simulink model "gm_uz_pmsm_model_9ph_21b_all_double"  (R2021b)
settings: Solver=FixedStepAuto  StartTime=0.0  StopTime=0.8  RelTol=1e-3
PreLoadFcn:
  | uz_pmsm_model_9ph_init_parameter
undefined symbols (not defined in the file or in its folder): a, b, c, friction_coefficient, inertia, k_i_d, k_i_q, k_p_d, k_p_q, Kpd, L_d, L_o1, L_o2, L_q, L_x1, L_x2, L_y1, L_y2, L_zero, polepair, psi_pm, R_1, static_friction_torque, Tnd, ts
libraries: hdlsllib x90, simulink x32, hdlmdlgenlib x17, dspsigops x7, slpidlib x2, spsAlphaBetaZerotodq0Lib x1, pid_lib x1, spsdq0toAlphaBetaZeroLib x1
(part 3 of 6)

== system gm_uz_pmsm_model_9ph_21b_all_double/uz_pmsm_model_9ph/dq_model_9ph/Wrapped State DTI ==
  note: https://de.mathworks.com/help/releases/R2021a/hdlcoder/ug/troubleshoot-generate-implementation-model-from-simscape-pmsm.html?searchHighlight=troubleshoot-generate-implementation-model-from-simscape-pmsm&s_tid=doc_srchtitle
  Angular Speed : Inport
  polepair : Inport  Port=2
  reset : Inport  Port=3
  Compare To Constant : simulink/Logic and Bit Operations/Compare To Constant  relop=>=  const=single(pi)  OutDataTypeStr=boolean
  Compare To Constant1 : simulink/Logic and Bit Operations/Compare To Constant  relop=<  const=single(-pi)  OutDataTypeStr=boolean
  Constant : Constant  Value=double(2*pi)  SampleTime=-1
  Delay1 : Delay  DelayLength=1  ExternalReset=Level
      settings: InputPortMap=u0,r5
  Gain : Gain  Gain=ts
  Product : Product
  Sum : Sum  Inputs=|++
  Sum1 : Sum  Inputs=|-+
  Sum2 : Sum  Inputs=|++
  Switch : Switch  Criteria=u2 > Threshold
  Switch1 : Switch  Criteria=u2 > Threshold
  Angular Position : Outport
  wires:
  Compare To Constant1/1 -> Switch1/2
  Delay1/1 -> Sum/1, Angular Position/1
  Constant/1 -> Sum2/1, Sum1/1
  Sum2/1 -> Switch1/1
  Switch1/1 -> Delay1/1  "Angular Position"
  Switch/1 -> Sum2/2, Compare To Constant1/1, Switch1/3
  Compare To Constant/1 -> Switch/2
  Sum/1 -> Compare To Constant/1, Sum1/2, Switch/3
  Sum1/1 -> Switch/1
  Gain/1 -> Sum/2
  reset/1 -> Delay1/2
  Product/1 -> Gain/1
  Angular Speed/1 -> Product/1
  polepair/1 -> Product/2

== system gm_uz_pmsm_model_9ph_21b_all_double/uz_pmsm_model_9ph/dq_model_9ph/mechanical_system ==
  note: load torque negative!!!
  note: This delay breaks the algebraic loop between mechanical and electrical system.
      | Introduces a delay of 500ns.
  reset : Inport
  M_Mi : Inport  Port=2
  reciprocal_J : Inport  Port=3
  load_torque : Inport  Port=4
  Delay : Delay  DelayLength=1
  Product11 : Product
  Sum1 : Sum  Inputs=|++
  integrator : Subsystem
  omega_mech : Outport
  wires:
  reciprocal_J/1 -> Product11/1
  Sum1/1 -> Product11/2
  load_torque/1 -> Sum1/2
  M_Mi/1 -> Delay/1
  Delay/1 -> Sum1/1
  integrator/1(outt) -> omega_mech/1
  Product11/1 -> integrator/1(in)
  reset/1 -> integrator/2(reset)

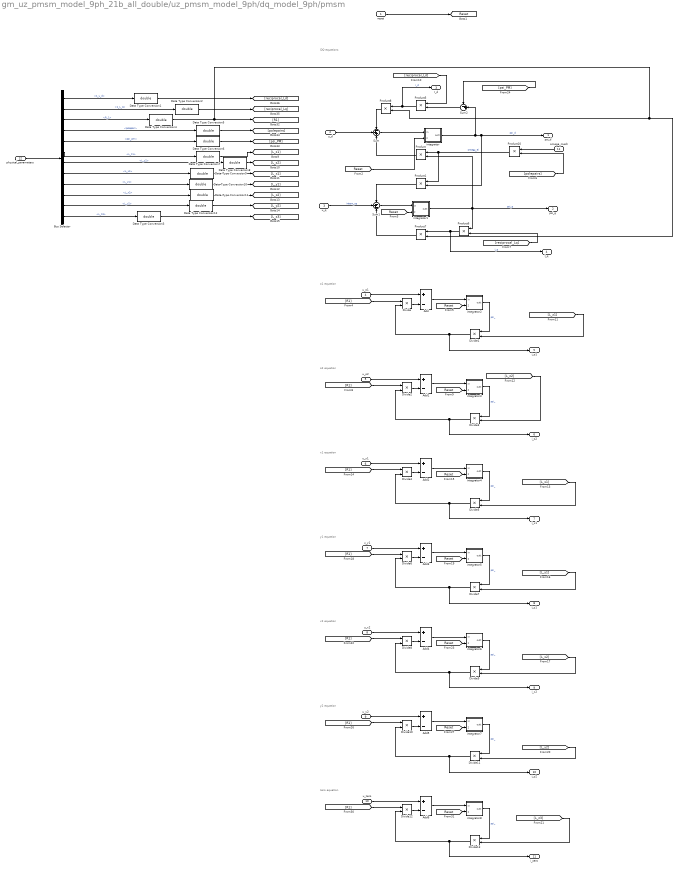
== system gm_uz_pmsm_model_9ph_21b_all_double/uz_pmsm_model_9ph/dq_model_9ph/pmsm ==
  note: o1 equation
  note: DQ equations
  note: o2 equation
  note: x1 equation
  note: y1 equation
  note: x2 equation
  note: y2 equation
  note: zero equation
  reset : Inport
  u_d : Inport  Port=2
  u_q : Inport  Port=3
  u_o1 : Inport  Port=4
  u_o2 : Inport  Port=5
  u_x1 : Inport  Port=6
  u_y1 : Inport  Port=7
  u_x2 : Inport  Port=8
  u_y2 : Inport  Port=9
  u_zero : Inport  Port=10
  omega_mech : Inport  Port=11
  physical_parameters : Inport  Port=12
  Add{,1..6} (7 alike) : Sum  Inputs=+-
  Bus Selector : BusSelector  OutputSignals=1_L_d,1_L_q,R_1,polepair,psi_pm,L_z1,L_z2,L_x1,L_y1,L_x2,L_y2,L_z3
  Data Type Conversion{1..12} (12 alike) : DataTypeConversion  OutDataTypeStr=double  RndMeth=Nearest
  Divide{,1..13} (14 alike) : Product  Inputs=**
  Product{,1,5..8,10} (7 alike) : Product
  Sum : Sum  Inputs=-++
  Sum1 : Sum  Inputs=-+-
  Sum2 : Sum  Inputs=-+|
  integrator : Subsystem
  integrator1 : Subsystem
  integrator2 : Subsystem
  integrator3 : Subsystem
  integrator4 : Subsystem
  integrator5 : Subsystem
  integrator6 : Subsystem
  integrator7 : Subsystem
  integrator8 : Subsystem
  psi_d : Outport
  psi_q : Outport  Port=2
  I_d : Outport  Port=3
  I_q : Outport  Port=4
  i_o1 : Outport  Port=5
  i_o2 : Outport  Port=6
  i_x1 : Outport  Port=7
  i_y1 : Outport  Port=8
  i_x2 : Outport  Port=9
  i_y2 : Outport  Port=10
  i_zero : Outport  Port=11
  tag scope: Reset=global
  wires:
  omega_mech/1 -> Product10/1
  u_q/1 -> Sum1/2  "intern_uq"
  Product/1 -> Sum/3
  Product5/1 -> I_d/1, Product8/1  "I_d"
  [reciprocal_Ld] -> Product5/1
  integrator1/1(outt) -> psi_q/1, Product/2, Product6/1  "psi_q"
  Product1/1 -> Sum1/1
  [psi_PM] -> Sum2/1
  Product6/1 -> I_q/1, Product7/1  "I_q"
  Product10/1 -> Product1/1, Product/1  "omega_el"
  integrator/1(outt) -> Sum2/2, psi_d/1, Product1/2  "psi_d"
  Sum2/1 -> Product5/2
  Product8/1 -> Sum/1
  [reciprocal_Lq] -> Product6/2
  Product7/1 -> Sum1/3
  reset/1 -> [Reset]
  [Reset] -> integrator/2(reset)
  [Reset] -> integrator1/2(reset)
  [Reset] -> integrator2/2(reset)
  [L_z1] -> Divide1/2
  u_o1/1 -> Add/1
  Divide1/1 -> i_o1/1, Divide/2
  Divide/1 -> Add/2
  [R1] -> Divide/1
  integrator2/1(outt) -> Divide1/1  "psi_"
  integrator3/1(outt) -> Divide3/1  "psi_"
  [R1] -> Divide2/1
  Divide2/1 -> Add1/2
  Divide3/1 -> i_o2/1, Divide2/2
  u_o2/1 -> Add1/1
  [L_z2] -> Divide3/2
  [Reset] -> integrator3/2(reset)
  [Reset] -> integrator4/2(reset)
  u_x1/1 -> Add2/1
  Divide5/1 -> i_x1/1, Divide4/2
  Divide4/1 -> Add2/2
  [R1] -> Divide4/1
  integrator4/1(outt) -> Divide5/1  "psi_"
  integrator5/1(outt) -> Divide7/1  "psi_"
  [R1] -> Divide6/1
  Divide6/1 -> Add3/2
  Divide7/1 -> i_y1/1, Divide6/2
  u_y1/1 -> Add3/1
  [Reset] -> integrator5/2(reset)
  [Reset] -> integrator6/2(reset)
  u_x2/1 -> Add4/1
  Divide9/1 -> i_x2/1, Divide8/2
  Divide8/1 -> Add4/2
  [R1] -> Divide8/1
  integrator6/1(outt) -> Divide9/1  "psi_"
  integrator7/1(outt) -> Divide11/1  "psi_"
  [R1] -> Divide10/1
  Divide10/1 -> Add5/2
  Divide11/1 -> i_y2/1, Divide10/2
  u_y2/1 -> Add5/1
  [Reset] -> integrator7/2(reset)
  [Reset] -> integrator8/2(reset)
  u_zero/1 -> Add6/1
  Divide13/1 -> i_zero/1, Divide12/2
  Divide12/1 -> Add6/2
  [R1] -> Divide12/1
  integrator8/1(outt) -> Divide13/1  "psi_"
  Bus Selector/1 -> Data Type Conversion1/1  "<1_L_d>"
  Bus Selector/4 -> Data Type Conversion5/1  "<polepair>"
  Bus Selector/8 -> Data Type Conversion9/1  "<L_x1>"
  Bus Selector/2 -> Data Type Conversion2/1  "<1_L_q>"
  Bus Selector/5 -> Data Type Conversion6/1  "<psi_pm>"
  Bus Selector/6 -> Data Type Conversion7/1  "<L_z1>"
  Bus Selector/7 -> Data Type Conversion8/1  "<L_z2>"
  Bus Selector/11 -> Data Type Conversion12/1  "<L_y2>"
  Bus Selector/3 -> Data Type Conversion4/1  "<R_1>"
  Bus Selector/10 -> Data Type Conversion11/1  "<L_x2>"
  physical_parameters/1 -> Bus Selector/1
  Bus Selector/9 -> Data Type Conversion10/1  "<L_y1>"
  [polepairs] -> Product10/2
  [L_x1] -> Divide5/2
  [L_y1] -> Divide7/2
  [L_x2] -> Divide9/2
  [L_y2] -> Divide11/2
  [L_z3] -> Divide13/2
  Sum/1 -> integrator/1(in)
  Sum1/1 -> integrator1/1(in)
  Add/1 -> integrator2/1(in)
  Add1/1 -> integrator3/1(in)
  Add2/1 -> integrator4/1(in)
  Add3/1 -> integrator5/1(in)
  Add4/1 -> integrator6/1(in)
  Add5/1 -> integrator7/1(in)
  Add6/1 -> integrator8/1(in)
  u_d/1 -> Sum/2
  Data Type Conversion1/1 -> [reciprocal_Ld]
  Data Type Conversion3/1 -> [L_z3]
  Bus Selector/12 -> Data Type Conversion3/1  "<L_z3>"
  Data Type Conversion2/1 -> [reciprocal_Lq]
  Data Type Conversion4/1 -> [R1], Product7/2, Product8/2
  Data Type Conversion5/1 -> [polepairs]
  Data Type Conversion6/1 -> [psi_PM]
  Data Type Conversion7/1 -> [L_z1]
  Data Type Conversion8/1 -> [L_z2]
  Data Type Conversion9/1 -> [L_x1]
  Data Type Conversion10/1 -> [L_y1]
  Data Type Conversion11/1 -> [L_x2]
  Data Type Conversion12/1 -> [L_y2]

== system gm_uz_pmsm_model_9ph_21b_all_double/uz_pmsm_model_9ph/dq_model_9ph/torque_calculation ==
  I_d : Inport
  I_q : Inport  Port=2
  psi_d : Inport  Port=3
  psi_q : Inport  Port=4
  polepairs : Inport  Port=5
  Factor : Gain  Gain=9/2
  Product2 : Product
  Product3 : Product
  Product9 : Product
  Sum3 : Sum  Inputs=-|+
  M_Mi : Outport
  wires:
  Sum3/1 -> Factor/1
  Product3/1 -> Sum3/2
  Product2/1 -> Sum3/1
  psi_q/1 -> Product2/2
  psi_d/1 -> Product3/1
  I_d/1 -> Product2/1
  I_q/1 -> Product3/2
  Product9/1 -> M_Mi/1  "M_Mi"
  polepairs/1 -> Product9/2
  Factor/1 -> Product9/1  "M_Mi"

== system gm_uz_pmsm_model_9ph_21b_all_double/uz_pmsm_model_9ph/abc_to_dq/abc_to_dq/Divide ==
  in0 : Inport  OutDataTypeStr=fixdt(1, 17, 15)  SampleTime=1e-08
  in1 : Inport  Port=2  OutDataTypeStr=fixdt(1, 25, 12)  SampleTime=1e-08
  globalSchedule : EnablePort  OutDataTypeStr=boolean
  Divide : Product  Inputs=**  OutDataTypeStr=fixdt(1, 25, 12)  SampleTime=1e-08
  HwModeRegister : Delay  DelayLength=double(1)  InitialCondition=0
  HwModeRegister1 : Delay  DelayLength=double(1)  InitialCondition=0
  PipelineRegister : Delay  DelayLength=double(1)  InitialCondition=0
  out0 : Outport  OutDataTypeStr=fixdt(1, 25, 12)  SampleTime=1e-08  InitialOutput=0
  wires:
  PipelineRegister/1 -> out0/1
  in0/1 -> HwModeRegister/1
  in1/1 -> HwModeRegister1/1
  Divide/1 -> PipelineRegister/1
  HwModeRegister/1 -> Divide/1
  HwModeRegister1/1 -> Divide/2

== system gm_uz_pmsm_model_9ph_21b_all_double/uz_pmsm_model_9ph/abc_to_dq/abc_to_dq/Divide1 ==
  in0 : Inport  OutDataTypeStr=fixdt(1, 17, 15)  SampleTime=1e-08
  in1 : Inport  Port=2  OutDataTypeStr=fixdt(1, 25, 12)  SampleTime=1e-08
  globalSchedule : EnablePort  OutDataTypeStr=boolean
  Divide1 : Product  Inputs=**  OutDataTypeStr=fixdt(1, 25, 12)  SampleTime=1e-08
  HwModeRegister : Delay  DelayLength=double(1)  InitialCondition=0
  HwModeRegister1 : Delay  DelayLength=double(1)  InitialCondition=0
  PipelineRegister : Delay  DelayLength=double(1)  InitialCondition=0
  out0 : Outport  OutDataTypeStr=fixdt(1, 25, 12)  SampleTime=1e-08  InitialOutput=0
  wires:
  PipelineRegister/1 -> out0/1
  in0/1 -> HwModeRegister/1
  in1/1 -> HwModeRegister1/1
  Divide1/1 -> PipelineRegister/1
  HwModeRegister/1 -> Divide1/1
  HwModeRegister1/1 -> Divide1/2

== system gm_uz_pmsm_model_9ph_21b_all_double/uz_pmsm_model_9ph/abc_to_dq/abc_to_dq/Divide11 ==
  in0 : Inport  OutDataTypeStr=fixdt(1, 17, 15)  SampleTime=1e-08
  in1 : Inport  Port=2  OutDataTypeStr=fixdt(1, 25, 12)  SampleTime=1e-08
  globalSchedule : EnablePort  OutDataTypeStr=boolean
  Divide1 : Product  Inputs=**  OutDataTypeStr=fixdt(1, 25, 12)  SampleTime=1e-08
  HwModeRegister : Delay  DelayLength=double(1)  InitialCondition=0
  HwModeRegister1 : Delay  DelayLength=double(1)  InitialCondition=0
  PipelineRegister : Delay  DelayLength=double(1)  InitialCondition=0
  out0 : Outport  OutDataTypeStr=fixdt(1, 25, 12)  SampleTime=1e-08  InitialOutput=0
  wires:
  PipelineRegister/1 -> out0/1
  in0/1 -> HwModeRegister/1
  in1/1 -> HwModeRegister1/1
  Divide1/1 -> PipelineRegister/1
  HwModeRegister/1 -> Divide1/1
  HwModeRegister1/1 -> Divide1/2

== system gm_uz_pmsm_model_9ph_21b_all_double/uz_pmsm_model_9ph/abc_to_dq/abc_to_dq/Divide2 ==
  in0 : Inport  OutDataTypeStr=fixdt(1, 17, 15)  SampleTime=1e-08
  in1 : Inport  Port=2  OutDataTypeStr=fixdt(1, 25, 12)  SampleTime=1e-08
  globalSchedule : EnablePort  OutDataTypeStr=boolean
  Divide2 : Product  Inputs=**  OutDataTypeStr=fixdt(1, 25, 12)  SampleTime=1e-08
  HwModeRegister : Delay  DelayLength=double(1)  InitialCondition=0
  HwModeRegister1 : Delay  DelayLength=double(1)  InitialCondition=0
  PipelineRegister : Delay  DelayLength=double(1)  InitialCondition=0
  out0 : Outport  OutDataTypeStr=fixdt(1, 25, 12)  SampleTime=1e-08  InitialOutput=0
  wires:
  PipelineRegister/1 -> out0/1
  in0/1 -> HwModeRegister/1
  in1/1 -> HwModeRegister1/1
  Divide2/1 -> PipelineRegister/1
  HwModeRegister/1 -> Divide2/1
  HwModeRegister1/1 -> Divide2/2

== system gm_uz_pmsm_model_9ph_21b_all_double/uz_pmsm_model_9ph/abc_to_dq/abc_to_dq/Divide21 ==
  in0 : Inport  OutDataTypeStr=fixdt(1, 17, 15)  SampleTime=1e-08
  in1 : Inport  Port=2  OutDataTypeStr=fixdt(1, 25, 12)  SampleTime=1e-08
  globalSchedule : EnablePort  OutDataTypeStr=boolean
  Divide2 : Product  Inputs=**  OutDataTypeStr=fixdt(1, 25, 12)  SampleTime=1e-08
  HwModeRegister : Delay  DelayLength=double(1)  InitialCondition=0
  HwModeRegister1 : Delay  DelayLength=double(1)  InitialCondition=0
  PipelineRegister : Delay  DelayLength=double(1)  InitialCondition=0
  out0 : Outport  OutDataTypeStr=fixdt(1, 25, 12)  SampleTime=1e-08  InitialOutput=0
  wires:
  PipelineRegister/1 -> out0/1
  in0/1 -> HwModeRegister/1
  in1/1 -> HwModeRegister1/1
  Divide2/1 -> PipelineRegister/1
  HwModeRegister/1 -> Divide2/1
  HwModeRegister1/1 -> Divide2/2

== system gm_uz_pmsm_model_9ph_21b_all_double/uz_pmsm_model_9ph/abc_to_dq/abc_to_dq/Divide3 ==
  in0 : Inport  OutDataTypeStr=fixdt(1, 17, 15)  SampleTime=1e-08
  in1 : Inport  Port=2  OutDataTypeStr=fixdt(1, 25, 12)  SampleTime=1e-08
  globalSchedule : EnablePort  OutDataTypeStr=boolean
  Divide3 : Product  Inputs=**  OutDataTypeStr=fixdt(1, 25, 12)  SampleTime=1e-08
  HwModeRegister : Delay  DelayLength=double(1)  InitialCondition=0
  HwModeRegister1 : Delay  DelayLength=double(1)  InitialCondition=0
  PipelineRegister : Delay  DelayLength=double(1)  InitialCondition=0
  out0 : Outport  OutDataTypeStr=fixdt(1, 25, 12)  SampleTime=1e-08  InitialOutput=0
  wires:
  PipelineRegister/1 -> out0/1
  in0/1 -> HwModeRegister/1
  in1/1 -> HwModeRegister1/1
  Divide3/1 -> PipelineRegister/1
  HwModeRegister/1 -> Divide3/1
  HwModeRegister1/1 -> Divide3/2

== system gm_uz_pmsm_model_9ph_21b_all_double/uz_pmsm_model_9ph/abc_to_dq/abc_to_dq/Divide31 ==
  in0 : Inport  OutDataTypeStr=fixdt(1, 17, 15)  SampleTime=1e-08
  in1 : Inport  Port=2  OutDataTypeStr=fixdt(1, 25, 12)  SampleTime=1e-08
  globalSchedule : EnablePort  OutDataTypeStr=boolean
  Divide3 : Product  Inputs=**  OutDataTypeStr=fixdt(1, 25, 12)  SampleTime=1e-08
  HwModeRegister : Delay  DelayLength=double(1)  InitialCondition=0
  HwModeRegister1 : Delay  DelayLength=double(1)  InitialCondition=0
  PipelineRegister : Delay  DelayLength=double(1)  InitialCondition=0
  out0 : Outport  OutDataTypeStr=fixdt(1, 25, 12)  SampleTime=1e-08  InitialOutput=0
  wires:
  PipelineRegister/1 -> out0/1
  in0/1 -> HwModeRegister/1
  in1/1 -> HwModeRegister1/1
  Divide3/1 -> PipelineRegister/1
  HwModeRegister/1 -> Divide3/1
  HwModeRegister1/1 -> Divide3/2

== system gm_uz_pmsm_model_9ph_21b_all_double/uz_pmsm_model_9ph/abc_to_dq/abc_to_dq/Divide4 ==
  in0 : Inport  OutDataTypeStr=fixdt(1, 17, 15)  SampleTime=1e-08
  in1 : Inport  Port=2  OutDataTypeStr=fixdt(1, 25, 12)  SampleTime=1e-08
  globalSchedule : EnablePort  OutDataTypeStr=boolean
  Divide : Product  Inputs=**  OutDataTypeStr=fixdt(1, 25, 12)  SampleTime=1e-08
  HwModeRegister : Delay  DelayLength=double(1)  InitialCondition=0
  HwModeRegister1 : Delay  DelayLength=double(1)  InitialCondition=0
  PipelineRegister : Delay  DelayLength=double(1)  InitialCondition=0
  out0 : Outport  OutDataTypeStr=fixdt(1, 25, 12)  SampleTime=1e-08  InitialOutput=0
  wires:
  PipelineRegister/1 -> out0/1
  in0/1 -> HwModeRegister/1
  in1/1 -> HwModeRegister1/1
  Divide/1 -> PipelineRegister/1
  HwModeRegister/1 -> Divide/1
  HwModeRegister1/1 -> Divide/2

== system gm_uz_pmsm_model_9ph_21b_all_double/uz_pmsm_model_9ph/abc_to_dq/abc_to_dq/Gain ==
  in0 : Inport  OutDataTypeStr=fixdt(1, 18, 19)  SampleTime=1e-08
  in1 : Inport  Port=2  OutDataTypeStr=fixdt(1, 18, 14)  SampleTime=1e-08
  globalSchedule : EnablePort  OutDataTypeStr=boolean
  Gain : Product  Inputs=**  OutDataTypeStr=fixdt(1, 18, 16)  SampleTime=1e-08
  HwModeRegister : Delay  DelayLength=double(1)  InitialCondition=0
  HwModeRegister1 : Delay  DelayLength=double(1)  InitialCondition=0
  PipelineRegister : Delay  DelayLength=double(1)  InitialCondition=0
  out0 : Outport  OutDataTypeStr=fixdt(1, 18, 16)  SampleTime=1e-08  InitialOutput=0
  wires:
  PipelineRegister/1 -> out0/1
  in0/1 -> HwModeRegister/1
  in1/1 -> HwModeRegister1/1
  Gain/1 -> PipelineRegister/1
  HwModeRegister/1 -> Gain/1
  HwModeRegister1/1 -> Gain/2

== system gm_uz_pmsm_model_9ph_21b_all_double/uz_pmsm_model_9ph/abc_to_dq/abc_to_dq/Gain2 ==
  in0 : Inport  OutDataTypeStr=fixdt(1, 25, 12)  PortDimensions=[3]  SampleTime=1e-08
  in1 : Inport  Port=2  OutDataTypeStr=fixdt(1, 18, 16)  SampleTime=1e-08
  globalSchedule : EnablePort  OutDataTypeStr=boolean
  Gain2 : Product  Inputs=**  OutDataTypeStr=fixdt(1, 43, 28)  SampleTime=1e-08
  HwModeRegister : Delay  DelayLength=double(1)  InitialCondition=0
  HwModeRegister1 : Delay  DelayLength=double(1)  InitialCondition=0
  PipelineRegister : Delay  DelayLength=double(1)  InitialCondition=0
  out0 : Outport  OutDataTypeStr=fixdt(1, 43, 28)  PortDimensions=[3]  SampleTime=1e-08  InitialOutput=0
  wires:
  PipelineRegister/1 -> out0/1
  in0/1 -> HwModeRegister/1
  in1/1 -> HwModeRegister1/1
  Gain2/1 -> PipelineRegister/1
  HwModeRegister/1 -> Gain2/1
  HwModeRegister1/1 -> Gain2/2

== system gm_uz_pmsm_model_9ph_21b_all_double/uz_pmsm_model_9ph/abc_to_dq/abc_to_dq/Gain21 ==
  in0 : Inport  OutDataTypeStr=fixdt(1, 25, 12)  PortDimensions=[3]  SampleTime=1e-08
  in1 : Inport  Port=2  OutDataTypeStr=fixdt(1, 18, 16)  SampleTime=1e-08
  globalSchedule : EnablePort  OutDataTypeStr=boolean
  Gain2 : Product  Inputs=**  OutDataTypeStr=fixdt(1, 43, 28)  SampleTime=1e-08
  HwModeRegister : Delay  DelayLength=double(1)  InitialCondition=0
  HwModeRegister1 : Delay  DelayLength=double(1)  InitialCondition=0
  PipelineRegister : Delay  DelayLength=double(1)  InitialCondition=0
  out0 : Outport  OutDataTypeStr=fixdt(1, 43, 28)  PortDimensions=[3]  SampleTime=1e-08  InitialOutput=0
  wires:
  PipelineRegister/1 -> out0/1
  in0/1 -> HwModeRegister/1
  in1/1 -> HwModeRegister1/1
  Gain2/1 -> PipelineRegister/1
  HwModeRegister/1 -> Gain2/1
  HwModeRegister1/1 -> Gain2/2

== system gm_uz_pmsm_model_9ph_21b_all_double/uz_pmsm_model_9ph/abc_to_dq/abc_to_dq/Gain22 ==
  in0 : Inport  OutDataTypeStr=fixdt(1, 25, 12)  PortDimensions=[3]  SampleTime=1e-08
  in1 : Inport  Port=2  OutDataTypeStr=fixdt(1, 18, 16)  SampleTime=1e-08
  globalSchedule : EnablePort  OutDataTypeStr=boolean
  Gain2 : Product  Inputs=**  OutDataTypeStr=fixdt(1, 43, 28)  SampleTime=1e-08
  HwModeRegister : Delay  DelayLength=double(1)  InitialCondition=0
  HwModeRegister1 : Delay  DelayLength=double(1)  InitialCondition=0
  PipelineRegister : Delay  DelayLength=double(1)  InitialCondition=0
  out0 : Outport  OutDataTypeStr=fixdt(1, 43, 28)  PortDimensions=[3]  SampleTime=1e-08  InitialOutput=0
  wires:
  PipelineRegister/1 -> out0/1
  in0/1 -> HwModeRegister/1
  in1/1 -> HwModeRegister1/1
  Gain2/1 -> PipelineRegister/1
  HwModeRegister/1 -> Gain2/1
  HwModeRegister1/1 -> Gain2/2

== system gm_uz_pmsm_model_9ph_21b_all_double/uz_pmsm_model_9ph/abc_to_dq/abc_to_dq/MMul_dot_product ==
  in0 : Inport  OutDataTypeStr=fixdt(1, 18, 16)  PortDimensions=[9 1]  SampleTime=1e-08
  in1 : Inport  Port=2  OutDataTypeStr=fixdt(1, 25, 12)  PortDimensions=[9 1]  SampleTime=1e-08
  globalSchedule : EnablePort  OutDataTypeStr=boolean
  HwModeRegister : Delay  DelayLength=double(1)  InitialCondition=0
  HwModeRegister1 : Delay  DelayLength=double(1)  InitialCondition=0
  MMul_dot_product : Product  Inputs=**  OutDataTypeStr=fixdt(1, 43, 28)  SampleTime=1e-08
  PipelineRegister : Delay  DelayLength=double(1)  InitialCondition=0
  out0 : Outport  OutDataTypeStr=fixdt(1, 43, 28)  PortDimensions=[9 1]  SampleTime=1e-08  InitialOutput=0
  wires:
  PipelineRegister/1 -> out0/1
  in0/1 -> HwModeRegister/1
  in1/1 -> HwModeRegister1/1
  MMul_dot_product/1 -> PipelineRegister/1
  HwModeRegister/1 -> MMul_dot_product/1
  HwModeRegister1/1 -> MMul_dot_product/2

== system gm_uz_pmsm_model_9ph_21b_all_double/uz_pmsm_model_9ph/abc_to_dq/abc_to_dq/MMul_dot_product1 ==
  in0 : Inport  OutDataTypeStr=fixdt(1, 18, 16)  PortDimensions=[9 1]  SampleTime=1e-08
  in1 : Inport  Port=2  OutDataTypeStr=fixdt(1, 25, 12)  PortDimensions=[9 1]  SampleTime=1e-08
  globalSchedule : EnablePort  OutDataTypeStr=boolean
  HwModeRegister : Delay  DelayLength=double(1)  InitialCondition=0
  HwModeRegister1 : Delay  DelayLength=double(1)  InitialCondition=0
  MMul_dot_product : Product  Inputs=**  OutDataTypeStr=fixdt(1, 43, 28)  SampleTime=1e-08
  PipelineRegister : Delay  DelayLength=double(1)  InitialCondition=0
  out0 : Outport  OutDataTypeStr=fixdt(1, 43, 28)  PortDimensions=[9 1]  SampleTime=1e-08  InitialOutput=0
  wires:
  PipelineRegister/1 -> out0/1
  in0/1 -> HwModeRegister/1
  in1/1 -> HwModeRegister1/1
  MMul_dot_product/1 -> PipelineRegister/1
  HwModeRegister/1 -> MMul_dot_product/1
  HwModeRegister1/1 -> MMul_dot_product/2

== system gm_uz_pmsm_model_9ph_21b_all_double/uz_pmsm_model_9ph/abc_to_dq/abc_to_dq/MMul_dot_product2 ==
  in0 : Inport  OutDataTypeStr=fixdt(1, 18, 16)  PortDimensions=[9 1]  SampleTime=1e-08
  in1 : Inport  Port=2  OutDataTypeStr=fixdt(1, 25, 12)  PortDimensions=[9 1]  SampleTime=1e-08
  globalSchedule : EnablePort  OutDataTypeStr=boolean
  HwModeRegister : Delay  DelayLength=double(1)  InitialCondition=0
  HwModeRegister1 : Delay  DelayLength=double(1)  InitialCondition=0
  MMul_dot_product : Product  Inputs=**  OutDataTypeStr=fixdt(1, 43, 28)  SampleTime=1e-08
  PipelineRegister : Delay  DelayLength=double(1)  InitialCondition=0
  out0 : Outport  OutDataTypeStr=fixdt(1, 43, 28)  PortDimensions=[9 1]  SampleTime=1e-08  InitialOutput=0
  wires:
  PipelineRegister/1 -> out0/1
  in0/1 -> HwModeRegister/1
  in1/1 -> HwModeRegister1/1
  MMul_dot_product/1 -> PipelineRegister/1
  HwModeRegister/1 -> MMul_dot_product/1
  HwModeRegister1/1 -> MMul_dot_product/2

== system gm_uz_pmsm_model_9ph_21b_all_double/uz_pmsm_model_9ph/abc_to_dq/abc_to_dq/MMul_dot_product3 ==
  in0 : Inport  OutDataTypeStr=fixdt(1, 18, 16)  PortDimensions=[9 1]  SampleTime=1e-08
  in1 : Inport  Port=2  OutDataTypeStr=fixdt(1, 25, 12)  PortDimensions=[9 1]  SampleTime=1e-08
  globalSchedule : EnablePort  OutDataTypeStr=boolean
  HwModeRegister : Delay  DelayLength=double(1)  InitialCondition=0
  HwModeRegister1 : Delay  DelayLength=double(1)  InitialCondition=0
  MMul_dot_product : Product  Inputs=**  OutDataTypeStr=fixdt(1, 43, 28)  SampleTime=1e-08
  PipelineRegister : Delay  DelayLength=double(1)  InitialCondition=0
  out0 : Outport  OutDataTypeStr=fixdt(1, 43, 28)  PortDimensions=[9 1]  SampleTime=1e-08  InitialOutput=0
  wires:
  PipelineRegister/1 -> out0/1
  in0/1 -> HwModeRegister/1
  in1/1 -> HwModeRegister1/1
  MMul_dot_product/1 -> PipelineRegister/1
  HwModeRegister/1 -> MMul_dot_product/1
  HwModeRegister1/1 -> MMul_dot_product/2

== system gm_uz_pmsm_model_9ph_21b_all_double/uz_pmsm_model_9ph/abc_to_dq/abc_to_dq/MMul_dot_product4 ==
  in0 : Inport  OutDataTypeStr=fixdt(1, 18, 16)  PortDimensions=[9 1]  SampleTime=1e-08
  in1 : Inport  Port=2  OutDataTypeStr=fixdt(1, 25, 12)  PortDimensions=[9 1]  SampleTime=1e-08
  globalSchedule : EnablePort  OutDataTypeStr=boolean
  HwModeRegister : Delay  DelayLength=double(1)  InitialCondition=0
  HwModeRegister1 : Delay  DelayLength=double(1)  InitialCondition=0
  MMul_dot_product : Product  Inputs=**  OutDataTypeStr=fixdt(1, 43, 28)  SampleTime=1e-08
  PipelineRegister : Delay  DelayLength=double(1)  InitialCondition=0
  out0 : Outport  OutDataTypeStr=fixdt(1, 43, 28)  PortDimensions=[9 1]  SampleTime=1e-08  InitialOutput=0
  wires:
  PipelineRegister/1 -> out0/1
  in0/1 -> HwModeRegister/1
  in1/1 -> HwModeRegister1/1
  MMul_dot_product/1 -> PipelineRegister/1
  HwModeRegister/1 -> MMul_dot_product/1
  HwModeRegister1/1 -> MMul_dot_product/2

== system gm_uz_pmsm_model_9ph_21b_all_double/uz_pmsm_model_9ph/abc_to_dq/abc_to_dq/MMul_dot_product5 ==
  in0 : Inport  OutDataTypeStr=fixdt(1, 18, 16)  PortDimensions=[9 1]  SampleTime=1e-08
  in1 : Inport  Port=2  OutDataTypeStr=fixdt(1, 25, 12)  PortDimensions=[9 1]  SampleTime=1e-08
  globalSchedule : EnablePort  OutDataTypeStr=boolean
  HwModeRegister : Delay  DelayLength=double(1)  InitialCondition=0
  HwModeRegister1 : Delay  DelayLength=double(1)  InitialCondition=0
  MMul_dot_product : Product  Inputs=**  OutDataTypeStr=fixdt(1, 43, 28)  SampleTime=1e-08
  PipelineRegister : Delay  DelayLength=double(1)  InitialCondition=0
  out0 : Outport  OutDataTypeStr=fixdt(1, 43, 28)  PortDimensions=[9 1]  SampleTime=1e-08  InitialOutput=0
  wires:
  PipelineRegister/1 -> out0/1
  in0/1 -> HwModeRegister/1
  in1/1 -> HwModeRegister1/1
  MMul_dot_product/1 -> PipelineRegister/1
  HwModeRegister/1 -> MMul_dot_product/1
  HwModeRegister1/1 -> MMul_dot_product/2

== system gm_uz_pmsm_model_9ph_21b_all_double/uz_pmsm_model_9ph/abc_to_dq/abc_to_dq/Product ==
  in0 : Inport  OutDataTypeStr=fixdt(1, 25, 12)  SampleTime=1e-08
  in1 : Inport  Port=2  OutDataTypeStr=fixdt(1, 18, 16)  SampleTime=1e-08
  globalSchedule : EnablePort  OutDataTypeStr=boolean
  HwModeRegister : Delay  DelayLength=double(1)  InitialCondition=0
  HwModeRegister1 : Delay  DelayLength=double(1)  InitialCondition=0
  PipelineRegister : Delay  DelayLength=double(1)  InitialCondition=0
  Product : Product  Inputs=**  OutDataTypeStr=fixdt(1, 25, 12)  SampleTime=1e-08
  out0 : Outport  OutDataTypeStr=fixdt(1, 25, 12)  SampleTime=1e-08  InitialOutput=0
  wires:
  PipelineRegister/1 -> out0/1
  in0/1 -> HwModeRegister/1
  in1/1 -> HwModeRegister1/1
  Product/1 -> PipelineRegister/1
  HwModeRegister/1 -> Product/1
  HwModeRegister1/1 -> Product/2

== system gm_uz_pmsm_model_9ph_21b_all_double/uz_pmsm_model_9ph/abc_to_dq/abc_to_dq/Product1 ==
  in0 : Inport  OutDataTypeStr=fixdt(1, 25, 12)  SampleTime=1e-08
  in1 : Inport  Port=2  OutDataTypeStr=fixdt(1, 18, 16)  SampleTime=1e-08
  globalSchedule : EnablePort  OutDataTypeStr=boolean
  HwModeRegister : Delay  DelayLength=double(1)  InitialCondition=0
  HwModeRegister1 : Delay  DelayLength=double(1)  InitialCondition=0
  PipelineRegister : Delay  DelayLength=double(1)  InitialCondition=0
  Product : Product  Inputs=**  OutDataTypeStr=fixdt(1, 25, 12)  SampleTime=1e-08
  out0 : Outport  OutDataTypeStr=fixdt(1, 25, 12)  SampleTime=1e-08  InitialOutput=0
  wires:
  PipelineRegister/1 -> out0/1
  in0/1 -> HwModeRegister/1
  in1/1 -> HwModeRegister1/1
  Product/1 -> PipelineRegister/1
  HwModeRegister/1 -> Product/1
  HwModeRegister1/1 -> Product/2

== system gm_uz_pmsm_model_9ph_21b_all_double/uz_pmsm_model_9ph/abc_to_dq/abc_to_dq/Product10 ==
  in0 : Inport  OutDataTypeStr=fixdt(1, 25, 12)  SampleTime=1e-08
  in1 : Inport  Port=2  OutDataTypeStr=fixdt(1, 18, 16)  SampleTime=1e-08
  globalSchedule : EnablePort  OutDataTypeStr=boolean
  HwModeRegister : Delay  DelayLength=double(1)  InitialCondition=0
  HwModeRegister1 : Delay  DelayLength=double(1)  InitialCondition=0
  PipelineRegister : Delay  DelayLength=double(1)  InitialCondition=0
  Product : Product  Inputs=**  OutDataTypeStr=fixdt(1, 25, 12)  SampleTime=1e-08
  out0 : Outport  OutDataTypeStr=fixdt(1, 25, 12)  SampleTime=1e-08  InitialOutput=0
  wires:
  PipelineRegister/1 -> out0/1
  in0/1 -> HwModeRegister/1
  in1/1 -> HwModeRegister1/1
  Product/1 -> PipelineRegister/1
  HwModeRegister/1 -> Product/1
  HwModeRegister1/1 -> Product/2

== system gm_uz_pmsm_model_9ph_21b_all_double/uz_pmsm_model_9ph/abc_to_dq/abc_to_dq/Product11 ==
  in0 : Inport  OutDataTypeStr=fixdt(1, 25, 12)  SampleTime=1e-08
  in1 : Inport  Port=2  OutDataTypeStr=fixdt(1, 18, 16)  SampleTime=1e-08
  globalSchedule : EnablePort  OutDataTypeStr=boolean
  HwModeRegister : Delay  DelayLength=double(1)  InitialCondition=0
  HwModeRegister1 : Delay  DelayLength=double(1)  InitialCondition=0
  PipelineRegister : Delay  DelayLength=double(1)  InitialCondition=0
  Product : Product  Inputs=**  OutDataTypeStr=fixdt(1, 25, 12)  SampleTime=1e-08
  out0 : Outport  OutDataTypeStr=fixdt(1, 25, 12)  SampleTime=1e-08  InitialOutput=0
  wires:
  PipelineRegister/1 -> out0/1
  in0/1 -> HwModeRegister/1
  in1/1 -> HwModeRegister1/1
  Product/1 -> PipelineRegister/1
  HwModeRegister/1 -> Product/1
  HwModeRegister1/1 -> Product/2

== system gm_uz_pmsm_model_9ph_21b_all_double/uz_pmsm_model_9ph/abc_to_dq/abc_to_dq/Product2 ==
  in0 : Inport  OutDataTypeStr=fixdt(1, 25, 12)  SampleTime=1e-08
  in1 : Inport  Port=2  OutDataTypeStr=fixdt(1, 18, 16)  SampleTime=1e-08
  globalSchedule : EnablePort  OutDataTypeStr=boolean
  HwModeRegister : Delay  DelayLength=double(1)  InitialCondition=0
  HwModeRegister1 : Delay  DelayLength=double(1)  InitialCondition=0
  PipelineRegister : Delay  DelayLength=double(1)  InitialCondition=0
  Product : Product  Inputs=**  OutDataTypeStr=fixdt(1, 25, 12)  SampleTime=1e-08
  out0 : Outport  OutDataTypeStr=fixdt(1, 25, 12)  SampleTime=1e-08  InitialOutput=0
  wires:
  PipelineRegister/1 -> out0/1
  in0/1 -> HwModeRegister/1
  in1/1 -> HwModeRegister1/1
  Product/1 -> PipelineRegister/1
  HwModeRegister/1 -> Product/1
  HwModeRegister1/1 -> Product/2

== system gm_uz_pmsm_model_9ph_21b_all_double/uz_pmsm_model_9ph/abc_to_dq/abc_to_dq/Product3 ==
  in0 : Inport  OutDataTypeStr=fixdt(1, 25, 12)  SampleTime=1e-08
  in1 : Inport  Port=2  OutDataTypeStr=fixdt(1, 18, 16)  SampleTime=1e-08
  globalSchedule : EnablePort  OutDataTypeStr=boolean
  HwModeRegister : Delay  DelayLength=double(1)  InitialCondition=0
  HwModeRegister1 : Delay  DelayLength=double(1)  InitialCondition=0
  PipelineRegister : Delay  DelayLength=double(1)  InitialCondition=0
  Product : Product  Inputs=**  OutDataTypeStr=fixdt(1, 25, 12)  SampleTime=1e-08
  out0 : Outport  OutDataTypeStr=fixdt(1, 25, 12)  SampleTime=1e-08  InitialOutput=0
  wires:
  PipelineRegister/1 -> out0/1
  in0/1 -> HwModeRegister/1
  in1/1 -> HwModeRegister1/1
  Product/1 -> PipelineRegister/1
  HwModeRegister/1 -> Product/1
  HwModeRegister1/1 -> Product/2

== system gm_uz_pmsm_model_9ph_21b_all_double/uz_pmsm_model_9ph/abc_to_dq/abc_to_dq/Product4 ==
  in0 : Inport  OutDataTypeStr=fixdt(1, 25, 12)  SampleTime=1e-08
  in1 : Inport  Port=2  OutDataTypeStr=fixdt(1, 18, 16)  SampleTime=1e-08
  globalSchedule : EnablePort  OutDataTypeStr=boolean
  HwModeRegister : Delay  DelayLength=double(1)  InitialCondition=0
  HwModeRegister1 : Delay  DelayLength=double(1)  InitialCondition=0
  PipelineRegister : Delay  DelayLength=double(1)  InitialCondition=0
  Product : Product  Inputs=**  OutDataTypeStr=fixdt(1, 25, 12)  SampleTime=1e-08
  out0 : Outport  OutDataTypeStr=fixdt(1, 25, 12)  SampleTime=1e-08  InitialOutput=0
  wires:
  PipelineRegister/1 -> out0/1
  in0/1 -> HwModeRegister/1
  in1/1 -> HwModeRegister1/1
  Product/1 -> PipelineRegister/1
  HwModeRegister/1 -> Product/1
  HwModeRegister1/1 -> Product/2

== system gm_uz_pmsm_model_9ph_21b_all_double/uz_pmsm_model_9ph/abc_to_dq/abc_to_dq/Product5 ==
  in0 : Inport  OutDataTypeStr=fixdt(1, 25, 12)  SampleTime=1e-08
  in1 : Inport  Port=2  OutDataTypeStr=fixdt(1, 18, 16)  SampleTime=1e-08
  globalSchedule : EnablePort  OutDataTypeStr=boolean
  HwModeRegister : Delay  DelayLength=double(1)  InitialCondition=0
  HwModeRegister1 : Delay  DelayLength=double(1)  InitialCondition=0
  PipelineRegister : Delay  DelayLength=double(1)  InitialCondition=0
  Product : Product  Inputs=**  OutDataTypeStr=fixdt(1, 25, 12)  SampleTime=1e-08
  out0 : Outport  OutDataTypeStr=fixdt(1, 25, 12)  SampleTime=1e-08  InitialOutput=0
  wires:
  PipelineRegister/1 -> out0/1
  in0/1 -> HwModeRegister/1
  in1/1 -> HwModeRegister1/1
  Product/1 -> PipelineRegister/1
  HwModeRegister/1 -> Product/1
  HwModeRegister1/1 -> Product/2

== system gm_uz_pmsm_model_9ph_21b_all_double/uz_pmsm_model_9ph/abc_to_dq/abc_to_dq/Product6 ==
  in0 : Inport  OutDataTypeStr=fixdt(1, 25, 12)  SampleTime=1e-08
  in1 : Inport  Port=2  OutDataTypeStr=fixdt(1, 18, 16)  SampleTime=1e-08
  globalSchedule : EnablePort  OutDataTypeStr=boolean
  HwModeRegister : Delay  DelayLength=double(1)  InitialCondition=0
  HwModeRegister1 : Delay  DelayLength=double(1)  InitialCondition=0
  PipelineRegister : Delay  DelayLength=double(1)  InitialCondition=0
  Product : Product  Inputs=**  OutDataTypeStr=fixdt(1, 25, 12)  SampleTime=1e-08
  out0 : Outport  OutDataTypeStr=fixdt(1, 25, 12)  SampleTime=1e-08  InitialOutput=0
  wires:
  PipelineRegister/1 -> out0/1
  in0/1 -> HwModeRegister/1
  in1/1 -> HwModeRegister1/1
  Product/1 -> PipelineRegister/1
  HwModeRegister/1 -> Product/1
  HwModeRegister1/1 -> Product/2

== system gm_uz_pmsm_model_9ph_21b_all_double/uz_pmsm_model_9ph/abc_to_dq/abc_to_dq/Product7 ==
  in0 : Inport  OutDataTypeStr=fixdt(1, 25, 12)  SampleTime=1e-08
  in1 : Inport  Port=2  OutDataTypeStr=fixdt(1, 18, 16)  SampleTime=1e-08
  globalSchedule : EnablePort  OutDataTypeStr=boolean
  HwModeRegister : Delay  DelayLength=double(1)  InitialCondition=0
  HwModeRegister1 : Delay  DelayLength=double(1)  InitialCondition=0
  PipelineRegister : Delay  DelayLength=double(1)  InitialCondition=0
  Product : Product  Inputs=**  OutDataTypeStr=fixdt(1, 25, 12)  SampleTime=1e-08
  out0 : Outport  OutDataTypeStr=fixdt(1, 25, 12)  SampleTime=1e-08  InitialOutput=0
  wires:
  PipelineRegister/1 -> out0/1
  in0/1 -> HwModeRegister/1
  in1/1 -> HwModeRegister1/1
  Product/1 -> PipelineRegister/1
  HwModeRegister/1 -> Product/1
  HwModeRegister1/1 -> Product/2

== system gm_uz_pmsm_model_9ph_21b_all_double/uz_pmsm_model_9ph/abc_to_dq/abc_to_dq/Product8 ==
  in0 : Inport  OutDataTypeStr=fixdt(1, 25, 12)  SampleTime=1e-08
  in1 : Inport  Port=2  OutDataTypeStr=fixdt(1, 18, 16)  SampleTime=1e-08
  globalSchedule : EnablePort  OutDataTypeStr=boolean
  HwModeRegister : Delay  DelayLength=double(1)  InitialCondition=0
  HwModeRegister1 : Delay  DelayLength=double(1)  InitialCondition=0
  PipelineRegister : Delay  DelayLength=double(1)  InitialCondition=0
  Product : Product  Inputs=**  OutDataTypeStr=fixdt(1, 25, 12)  SampleTime=1e-08
  out0 : Outport  OutDataTypeStr=fixdt(1, 25, 12)  SampleTime=1e-08  InitialOutput=0
  wires:
  PipelineRegister/1 -> out0/1
  in0/1 -> HwModeRegister/1
  in1/1 -> HwModeRegister1/1
  Product/1 -> PipelineRegister/1
  HwModeRegister/1 -> Product/1
  HwModeRegister1/1 -> Product/2

== system gm_uz_pmsm_model_9ph_21b_all_double/uz_pmsm_model_9ph/abc_to_dq/abc_to_dq/Product9 ==
  in0 : Inport  OutDataTypeStr=fixdt(1, 25, 12)  SampleTime=1e-08
  in1 : Inport  Port=2  OutDataTypeStr=fixdt(1, 18, 16)  SampleTime=1e-08
  globalSchedule : EnablePort  OutDataTypeStr=boolean
  HwModeRegister : Delay  DelayLength=double(1)  InitialCondition=0
  HwModeRegister1 : Delay  DelayLength=double(1)  InitialCondition=0
  PipelineRegister : Delay  DelayLength=double(1)  InitialCondition=0
  Product : Product  Inputs=**  OutDataTypeStr=fixdt(1, 25, 12)  SampleTime=1e-08
  out0 : Outport  OutDataTypeStr=fixdt(1, 25, 12)  SampleTime=1e-08  InitialOutput=0
  wires:
  PipelineRegister/1 -> out0/1
  in0/1 -> HwModeRegister/1
  in1/1 -> HwModeRegister1/1
  Product/1 -> PipelineRegister/1
  HwModeRegister/1 -> Product/1
  HwModeRegister1/1 -> Product/2

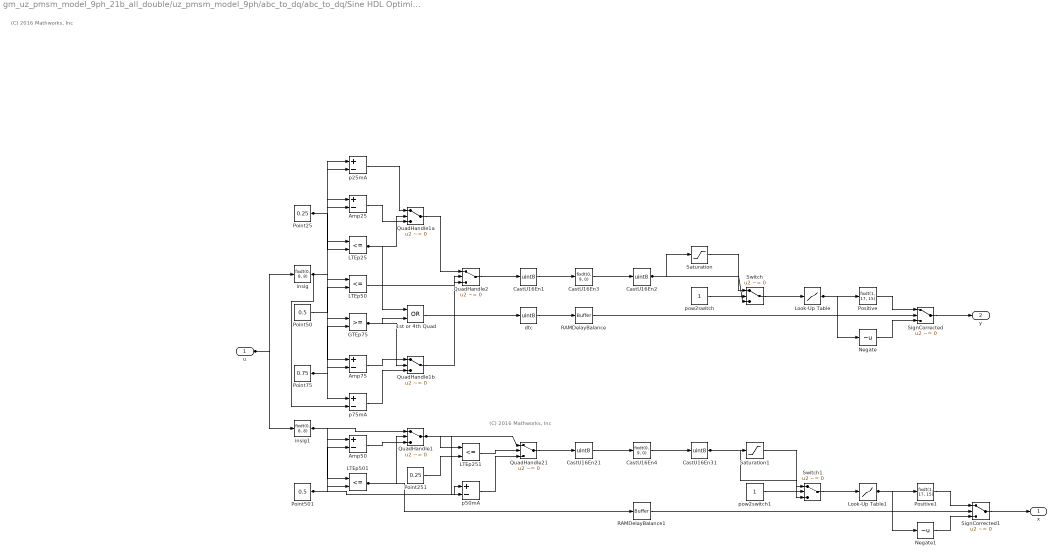
== system gm_uz_pmsm_model_9ph_21b_all_double/uz_pmsm_model_9ph/abc_to_dq/abc_to_dq/Sine HDL Optimized ==
  note: (C) 2016 Mathworks, Inc
  note: (C) 2016 Mathworks, Inc
  u : Inport  OutDataTypeStr=fixdt(1, 18, 16)  SampleTime=1e-08
  1st or 4th Quad : Logic  Operator=OR  AllPortsSameDT=off  OutDataTypeStr=boolean  SampleTime=1e-08
  Amp25 : Sum  Inputs=+-  AccumDataTypeStr=fixdt(1, 18, 17)  OutDataTypeStr=fixdt(1, 18, 17)  SampleTime=1e-08
  Amp50 : Sum  Inputs=+-  AccumDataTypeStr=fixdt(1, 18, 17)  OutDataTypeStr=fixdt(1, 18, 17)  SampleTime=1e-08
  Amp75 : Sum  Inputs=+-  AccumDataTypeStr=fixdt(1, 18, 17)  OutDataTypeStr=fixdt(1, 18, 17)  SampleTime=1e-08
  CastU16En1 : DataTypeConversion  OutDataTypeStr=uint8  ConvertRealWorld=Stored Integer (SI)  SampleTime=1e-08
  CastU16En2 : DataTypeConversion  OutDataTypeStr=uint8  ConvertRealWorld=Stored Integer (SI)  SampleTime=1e-08  SaturateOnIntegerOverflow=on
  CastU16En21 : DataTypeConversion  OutDataTypeStr=uint8  ConvertRealWorld=Stored Integer (SI)  SampleTime=1e-08
  CastU16En3 : DataTypeConversion  OutDataTypeStr=fixdt(0, 9, 0)  SampleTime=1e-08
  CastU16En31 : DataTypeConversion  OutDataTypeStr=uint8  ConvertRealWorld=Stored Integer (SI)  SampleTime=1e-08  SaturateOnIntegerOverflow=on
  CastU16En4 : DataTypeConversion  OutDataTypeStr=fixdt(0, 9, 0)  SampleTime=1e-08
  GTEp75 : RelationalOperator  OutDataTypeStr=boolean  SampleTime=1e-08  RndMeth=Nearest
  LTEp{25,50,251,501} (4 alike) : RelationalOperator  Operator=<=  OutDataTypeStr=boolean  SampleTime=1e-08  RndMeth=Nearest
  Look-Up Table : Lookup_n-D  NumberOfTableDimensions=1  BreakpointsForDimension1="fi(\"numerictype\",numerictype(0,8,0),\"fimath\",fimath(\"RoundingMethod\", \"Floor\",\"OverflowAction\", \"Wrap\",\"ProductMode\",\"FullPrecision\",\"SumMode\",\"FullPrecision\"),\"Value\",\"[0 1 2 3 4 5 6 7 8 9 10 11 12 13 14 15 16 17 18 19 20 21 22 23 24 25 26 27 28 29 30 31 32 33 34 35 36 37 38 39 40 41 42 43 44 45 46 47 48 49 50 51 52 53 54 55 56 57 58 59 60 61 62 63]\")"  Table="reshape(fi(\"numerictype\",numerictype(1,17,15),\"fimath\",fimath(\"RoundingMethod\", \"Floor\",\"OverflowAction\", \"Wrap\",\"ProductMode\",\"FullPrecision\",\"SumMode\",\"FullPrecision\"),\"Value\",\"[0;0.0245361328125;0.049072265625;0.073577880859375;0.0980224609375;0.122406005859375;0.146728515625;0.17095947265625;0.195098876953125;0.2191162109375;0.24298095703125;0.2667236328125;0.290283203125;0.313690185546875;0.336883544921875;0.359893798828125;0.3826904296875;0.405242919921875;0.42755126953125;0.449615478515625;0.471405029296875;0.492889404296875;0.51409912109375;0.535003662109375;0.555572509765625;0.5758056640625;0.595703125;0.615234375;0.6343994140625;0.653167724609375;0.67156982421875;0.689544677734375;0.70709228515625;0.7242431640625;0.740936279296875;0.7572021484375;0.77301025390625;0.788360595703125;0.80322265625;0.817596435546875;0.83148193359375;0.8448486328125;0.85772705078125;0.870086669921875;0.881927490234375;0.893218994140625;0.90399169921875;0.914215087890625;0.92388916015625;0.9329833984375;0.941558837890625;0.94952392578125;0.956939697265625;0.963775634765625;0.97003173828125;0.9757080078125;0.98077392578125;0.98529052734375;0.989166259765625;0.99249267578125;0.99517822265625;0.997283935546875;0.998809814453125;0.99969482421875]\"), [1  64])"  InterpMethod=Flat  ExtrapMethod=Clip  DiagnosticForOutOfRangeInput=Error  SampleTime=1e-08  OutDataTypeStr=fixdt(1, 17, 15)  InputSameDT=on
  Look-Up Table1 : Lookup_n-D  NumberOfTableDimensions=1  BreakpointsForDimension1="fi(\"numerictype\",numerictype(0,8,0),\"fimath\",fimath(\"RoundingMethod\", \"Floor\",\"OverflowAction\", \"Wrap\",\"ProductMode\",\"FullPrecision\",\"SumMode\",\"FullPrecision\"),\"Value\",\"[0 1 2 3 4 5 6 7 8 9 10 11 12 13 14 15 16 17 18 19 20 21 22 23 24 25 26 27 28 29 30 31 32 33 34 35 36 37 38 39 40 41 42 43 44 45 46 47 48 49 50 51 52 53 54 55 56 57 58 59 60 61 62 63]\")"  Table="reshape(fi(\"numerictype\",numerictype(1,17,15),\"fimath\",fimath(\"RoundingMethod\", \"Floor\",\"OverflowAction\", \"Wrap\",\"ProductMode\",\"FullPrecision\",\"SumMode\",\"FullPrecision\"),\"Value\",\"[0;0.0245361328125;0.049072265625;0.073577880859375;0.0980224609375;0.122406005859375;0.146728515625;0.17095947265625;0.195098876953125;0.2191162109375;0.24298095703125;0.2667236328125;0.290283203125;0.313690185546875;0.336883544921875;0.359893798828125;0.3826904296875;0.405242919921875;0.42755126953125;0.449615478515625;0.471405029296875;0.492889404296875;0.51409912109375;0.535003662109375;0.555572509765625;0.5758056640625;0.595703125;0.615234375;0.6343994140625;0.653167724609375;0.67156982421875;0.689544677734375;0.70709228515625;0.7242431640625;0.740936279296875;0.7572021484375;0.77301025390625;0.788360595703125;0.80322265625;0.817596435546875;0.83148193359375;0.8448486328125;0.85772705078125;0.870086669921875;0.881927490234375;0.893218994140625;0.90399169921875;0.914215087890625;0.92388916015625;0.9329833984375;0.941558837890625;0.94952392578125;0.956939697265625;0.963775634765625;0.97003173828125;0.9757080078125;0.98077392578125;0.98529052734375;0.989166259765625;0.99249267578125;0.99517822265625;0.997283935546875;0.998809814453125;0.99969482421875]\"), [1  64])"  InterpMethod=Flat  ExtrapMethod=Clip  DiagnosticForOutOfRangeInput=Error  SampleTime=1e-08  OutDataTypeStr=fixdt(1, 17, 15)  InputSameDT=on
  Negate : UnaryMinus  SampleTime=1e-08
  Negate1 : UnaryMinus  SampleTime=1e-08
  Point25 : Constant  Value=0.25  OutDataTypeStr=fixdt(0, 17, 17)  SampleTime=1e-08
  Point251 : Constant  Value=0.25  OutDataTypeStr=fixdt(0, 17, 17)  SampleTime=1e-08
  Point50 : Constant  Value=0.5  OutDataTypeStr=fixdt(0, 17, 17)  SampleTime=1e-08
  Point501 : Constant  Value=0.5  OutDataTypeStr=fixdt(0, 17, 17)  SampleTime=1e-08
  Point75 : Constant  Value=0.75  OutDataTypeStr=fixdt(0, 17, 17)  SampleTime=1e-08
  Positive : DataTypeConversion  OutDataTypeStr=fixdt(1, 17, 15)  SampleTime=1e-08
  Positive1 : DataTypeConversion  OutDataTypeStr=fixdt(1, 17, 15)  SampleTime=1e-08
  QuadHandle1 : Switch  Criteria=u2 ~= 0  Threshold=double(0)  OutDataTypeStr=fixdt(1, 18, 17)  SampleTime=1e-08
  QuadHandle1a : Switch  Criteria=u2 ~= 0  Threshold=double(0)  OutDataTypeStr=fixdt(1, 18, 17)  SampleTime=1e-08
  QuadHandle1b : Switch  Criteria=u2 ~= 0  Threshold=double(0)  OutDataTypeStr=fixdt(1, 18, 17)  SampleTime=1e-08
  QuadHandle2 : Switch  Criteria=u2 ~= 0  Threshold=double(0)  OutDataTypeStr=fixdt(0, 8, 8)  SampleTime=1e-08  SaturateOnIntegerOverflow=on
  QuadHandle21 : Switch  Criteria=u2 ~= 0  Threshold=double(0)  OutDataTypeStr=fixdt(0, 8, 8)  SampleTime=1e-08
  RAMDelayBalance : hdlmdlgenlib/Buffer
      settings: SourceProductBaseCode=SL
  RAMDelayBalance1 : hdlmdlgenlib/Buffer
      settings: SourceProductBaseCode=SL
  Saturation : Saturate  UpperLimit="fi(0,0,8,0,\"hex\",\"3f\")"  LowerLimit="fi(0,0,8,0,\"hex\",\"00\")"  SampleTime=1e-08  OutDataTypeStr=uint8
  Saturation1 : Saturate  UpperLimit="fi(0,0,8,0,\"hex\",\"3f\")"  LowerLimit="fi(0,0,8,0,\"hex\",\"00\")"  SampleTime=1e-08  OutDataTypeStr=uint8
  SignCorrected : Switch  Criteria=u2 ~= 0  Threshold=double(0)  OutDataTypeStr=fixdt(1, 17, 15)  SampleTime=1e-08
  SignCorrected1 : Switch  Criteria=u2 ~= 0  Threshold=double(0)  OutDataTypeStr=fixdt(1, 17, 15)  SampleTime=1e-08
  Switch : Switch  Criteria=u2 ~= 0  Threshold=double(0)  OutDataTypeStr=uint8  SampleTime=1e-08
  Switch1 : Switch  Criteria=u2 ~= 0  Threshold=double(0)  OutDataTypeStr=uint8  SampleTime=1e-08
  dtc : DataTypeConversion  OutDataTypeStr=uint8  SampleTime=1e-08
  insig : DataTypeConversion  OutDataTypeStr=fixdt(0, 8, 8)  SampleTime=1e-08
  insig1 : DataTypeConversion  OutDataTypeStr=fixdt(0, 8, 8)  SampleTime=1e-08
  p25mA : Sum  Inputs=+-  AccumDataTypeStr=fixdt(1, 18, 17)  OutDataTypeStr=fixdt(1, 18, 17)  SampleTime=1e-08
  p50mA : Sum  Inputs=+-  AccumDataTypeStr=fixdt(1, 19, 17)  OutDataTypeStr=fixdt(1, 19, 17)  SampleTime=1e-08
  p75mA : Sum  Inputs=+-  AccumDataTypeStr=fixdt(1, 18, 17)  OutDataTypeStr=fixdt(1, 18, 17)  SampleTime=1e-08
  pow2switch : Constant  OutDataTypeStr=boolean  SampleTime=1e-08
  pow2switch1 : Constant  OutDataTypeStr=boolean  SampleTime=1e-08
  x : Outport  SampleTime=1e-08
  y : Outport  Port=2  SampleTime=1e-08
  wires:
  dtc/1 -> RAMDelayBalance/1
  Amp25/1 -> QuadHandle1a/3
  Amp75/1 -> QuadHandle1b/1
  CastU16En1/1 -> CastU16En3/1
  CastU16En2/1 -> Switch/3, Saturation/1
  CastU16En3/1 -> CastU16En2/1
  GTEp75/1 -> QuadHandle1b/2, 1st or 4th Quad/2
  LTEp25/1 -> QuadHandle1a/2, 1st or 4th Quad/1
  LTEp50/1 -> QuadHandle2/2
  Look-Up Table/1 -> Positive/1, Negate/1
  Negate/1 -> SignCorrected/3
  Point25/1 -> p25mA/1, LTEp25/2, Amp25/2
  Point50/1 -> LTEp50/2
  Point75/1 -> p75mA/1, GTEp75/2, Amp75/2
  Positive/1 -> SignCorrected/1
  QuadHandle1a/1 -> QuadHandle2/1
  QuadHandle1b/1 -> QuadHandle2/3
  QuadHandle2/1 -> CastU16En1/1
  RAMDelayBalance/1 -> SignCorrected/2
  Saturation/1 -> Switch/1
  SignCorrected/1 -> y/1
  Switch/1 -> Look-Up Table/1
  insig/1 -> p75mA/2, p25mA/2, LTEp50/1, LTEp25/1, GTEp75/1, Amp75/1, Amp25/1
  p25mA/1 -> QuadHandle1a/1
  p75mA/1 -> QuadHandle1b/3
  pow2switch/1 -> Switch/2
  Amp50/1 -> QuadHandle1/3
  CastU16En21/1 -> CastU16En4/1
  CastU16En31/1 -> Switch1/3, Saturation1/1
  CastU16En4/1 -> CastU16En31/1
  LTEp251/1 -> QuadHandle21/2
  LTEp501/1 -> QuadHandle1/2, RAMDelayBalance1/1
  Look-Up Table1/1 -> Positive1/1, Negate1/1
  Negate1/1 -> SignCorrected1/3
  Point251/1 -> LTEp251/2
  Point501/1 -> p50mA/1, LTEp501/2, Amp50/2
  Positive1/1 -> SignCorrected1/1
  QuadHandle1/1 -> p50mA/2, QuadHandle21/1, LTEp251/1
  QuadHandle21/1 -> CastU16En21/1
  RAMDelayBalance1/1 -> SignCorrected1/2
  Saturation1/1 -> Switch1/1
  SignCorrected1/1 -> x/1
  Switch1/1 -> Look-Up Table1/1
  insig1/1 -> QuadHandle1/1, LTEp501/1, Amp50/1
  p50mA/1 -> QuadHandle21/3
  pow2switch1/1 -> Switch1/2
  1st or 4th Quad/1 -> dtc/1
  u/1 -> insig1/1, insig/1

== system gm_uz_pmsm_model_9ph_21b_all_double/uz_pmsm_model_9ph/abc_to_dq/abc_to_dq/_adder_MultiplyAdd ==
  in0 : Inport  OutDataTypeStr=fixdt(1, 18, 17)  SampleTime=1e-08
  in1 : Inport  Port=2  OutDataTypeStr=fixdt(1, 25, 12)  SampleTime=1e-08
  in2 : Inport  Port=3  OutDataTypeStr=fixdt(1, 25, 12)  SampleTime=1e-08
  globalSchedule : EnablePort  OutDataTypeStr=boolean
  HwModeRegister : Delay  DelayLength=double(1)  InitialCondition=0
  HwModeRegister1 : Delay  DelayLength=double(1)  InitialCondition=0
  HwModeRegister2 : Delay  DelayLength=double(1)  InitialCondition=0
  PipelineRegister : Delay  DelayLength=double(2)  InitialCondition=0
  _adder_MultiplyAdd : hdlsllib/HDL Operations/Multiply-Add  Function=c+(a.*b)  datatype=fixdt(1, 44, 29)  DoSatur=off  FMA=off
      settings: SourceProductBaseCode=SL
  out0 : Outport  OutDataTypeStr=fixdt(1, 44, 29)  SampleTime=1e-08  InitialOutput=0
  wires:
  PipelineRegister/1 -> out0/1
  in0/1 -> HwModeRegister/1
  in1/1 -> HwModeRegister1/1
  in2/1 -> HwModeRegister2/1
  _adder_MultiplyAdd/1 -> PipelineRegister/1
  HwModeRegister/1 -> _adder_MultiplyAdd/1
  HwModeRegister1/1 -> _adder_MultiplyAdd/2
  HwModeRegister2/1 -> _adder_MultiplyAdd/3

== system gm_uz_pmsm_model_9ph_21b_all_double/uz_pmsm_model_9ph/abc_to_dq/abc_to_dq/_adder_MultiplyAdd1 ==
  in0 : Inport  OutDataTypeStr=fixdt(1, 18, 17)  SampleTime=1e-08
  in1 : Inport  Port=2  OutDataTypeStr=fixdt(1, 25, 12)  SampleTime=1e-08
  in2 : Inport  Port=3  OutDataTypeStr=fixdt(1, 25, 12)  SampleTime=1e-08
  globalSchedule : EnablePort  OutDataTypeStr=boolean
  HwModeRegister : Delay  DelayLength=double(1)  InitialCondition=0
  HwModeRegister1 : Delay  DelayLength=double(1)  InitialCondition=0
  HwModeRegister2 : Delay  DelayLength=double(1)  InitialCondition=0
  PipelineRegister : Delay  DelayLength=double(2)  InitialCondition=0
  _adder_MultiplyAdd : hdlsllib/HDL Operations/Multiply-Add  Function=c+(a.*b)  datatype=fixdt(1, 44, 29)  DoSatur=off  FMA=off
      settings: SourceProductBaseCode=SL
  out0 : Outport  OutDataTypeStr=fixdt(1, 44, 29)  SampleTime=1e-08  InitialOutput=0
  wires:
  PipelineRegister/1 -> out0/1
  in0/1 -> HwModeRegister/1
  in1/1 -> HwModeRegister1/1
  in2/1 -> HwModeRegister2/1
  _adder_MultiplyAdd/1 -> PipelineRegister/1
  HwModeRegister/1 -> _adder_MultiplyAdd/1
  HwModeRegister1/1 -> _adder_MultiplyAdd/2
  HwModeRegister2/1 -> _adder_MultiplyAdd/3

== system gm_uz_pmsm_model_9ph_21b_all_double/uz_pmsm_model_9ph/abc_to_dq/abc_to_dq/_adder_MultiplyAdd10 ==
  in0 : Inport  OutDataTypeStr=fixdt(1, 18, 17)  SampleTime=1e-08
  in1 : Inport  Port=2  OutDataTypeStr=fixdt(1, 25, 12)  SampleTime=1e-08
  in2 : Inport  Port=3  OutDataTypeStr=fixdt(1, 25, 12)  SampleTime=1e-08
  globalSchedule : EnablePort  OutDataTypeStr=boolean
  HwModeRegister : Delay  DelayLength=double(1)  InitialCondition=0
  HwModeRegister1 : Delay  DelayLength=double(1)  InitialCondition=0
  HwModeRegister2 : Delay  DelayLength=double(1)  InitialCondition=0
  PipelineRegister : Delay  DelayLength=double(2)  InitialCondition=0
  _adder_MultiplyAdd : hdlsllib/HDL Operations/Multiply-Add  Function=c+(a.*b)  datatype=fixdt(1, 44, 29)  DoSatur=off  FMA=off
      settings: SourceProductBaseCode=SL
  out0 : Outport  OutDataTypeStr=fixdt(1, 44, 29)  SampleTime=1e-08  InitialOutput=0
  wires:
  PipelineRegister/1 -> out0/1
  in0/1 -> HwModeRegister/1
  in1/1 -> HwModeRegister1/1
  in2/1 -> HwModeRegister2/1
  _adder_MultiplyAdd/1 -> PipelineRegister/1
  HwModeRegister/1 -> _adder_MultiplyAdd/1
  HwModeRegister1/1 -> _adder_MultiplyAdd/2
  HwModeRegister2/1 -> _adder_MultiplyAdd/3

== system gm_uz_pmsm_model_9ph_21b_all_double/uz_pmsm_model_9ph/abc_to_dq/abc_to_dq/_adder_MultiplyAdd11 ==
  in0 : Inport  OutDataTypeStr=fixdt(1, 18, 17)  SampleTime=1e-08
  in1 : Inport  Port=2  OutDataTypeStr=fixdt(1, 25, 12)  SampleTime=1e-08
  in2 : Inport  Port=3  OutDataTypeStr=fixdt(1, 25, 12)  SampleTime=1e-08
  globalSchedule : EnablePort  OutDataTypeStr=boolean
  HwModeRegister : Delay  DelayLength=double(1)  InitialCondition=0
  HwModeRegister1 : Delay  DelayLength=double(1)  InitialCondition=0
  HwModeRegister2 : Delay  DelayLength=double(1)  InitialCondition=0
  PipelineRegister : Delay  DelayLength=double(2)  InitialCondition=0
  _adder_MultiplyAdd : hdlsllib/HDL Operations/Multiply-Add  Function=c+(a.*b)  datatype=fixdt(1, 44, 29)  DoSatur=off  FMA=off
      settings: SourceProductBaseCode=SL
  out0 : Outport  OutDataTypeStr=fixdt(1, 44, 29)  SampleTime=1e-08  InitialOutput=0
  wires:
  PipelineRegister/1 -> out0/1
  in0/1 -> HwModeRegister/1
  in1/1 -> HwModeRegister1/1
  in2/1 -> HwModeRegister2/1
  _adder_MultiplyAdd/1 -> PipelineRegister/1
  HwModeRegister/1 -> _adder_MultiplyAdd/1
  HwModeRegister1/1 -> _adder_MultiplyAdd/2
  HwModeRegister2/1 -> _adder_MultiplyAdd/3
